simulink model "RadioReceiver_FP_clean"  (R2017a)
settings: Solver=FixedStepDiscrete  StartTime=0.0  StopTime=10.0  RelTol=1e-3
InitFcn:
  | barker = comm.BarkerCode('SamplesPerFrame', 28, 'Length', 11);
  | seq = barker()+1;
  | M = 4;
  | hPSKModTrain   = comm.PSKModulator(M, ...
  |     'PhaseOffset',pi/4, ...
  |     'SymbolMapping','Binary');
  | xPreambleSeq = hPSKModTrain(seq);
  | 
  | 
  | %%%%%%%%%%%%
  | 
  | % AGC Preamble
  | reps = 5;
  | barker = comm.BarkerCode('SamplesPerFrame', 16, 'Length', 13);
  | seq = barker()+1;
  | %preamble = zeros(16*reps,1);
  | preambleFull = repmat(seq,reps,1);
  | rctFilt = comm.RaisedCosineTransmitFilter('FilterSpanInSymbols', 128,...
  | 'RolloffFactor',0.5,...
  | 'OutputSamplesPerSymbol',4);
  | preambleFullFilt = rctFilt(preambleFull);
  | 
  | %%%%%%%%%%%%
  | 
  | RadioSampleRate = 1e6;
  | RadioFrameLength = 1e5;
  | 
  | VibertiTracebackLength = 34+20;
  | numTrainingSamples = 250;
  | crc32Poly = [1 0 0 0 0 0 1 0 0 1 1 0 0 0 0 0 1 0 0 0 1 1 1 0 1 1 0 1 1 0 1 1 1];
  | crcDecodeLag = length(crc32Poly)+2;
  | 
  | %%%%%%%%%%%%
  | 
  | beta = 0.5;
  | span = 8;
  | sps = 4;
  | filterGain = 1;
  | coeff = rcosdesign(beta, span, sps, 'sqrt')*filterGain;
  | 
  | %%%%%%%%%%%%
  | 
  | samplesPerSymbol = 4;
  | maxPacketBits = 8*1500;
  | bItsPerSymbol = 2;
  | CodeRate = 2;
  | tailSymbols = 40;
  | maxPayloadSymbols = maxPacketBits*CodeRate/bItsPerSymbol+tailSymbols;
undefined symbols (not defined in the file or in its folder): F, j
libraries: dsphdlfiltering x20, simulink x7, dspstat3 x2, hdlsllib x2, commdigbbndpm3 x2, commsource2 x1, commcrc2 x1, commseqgen3 x1, commcnvcod2 x1, commutil2 x1, zc706fmc234_lib x1
(part 1 of 3)
settings Model: DataTypeOverride=Off  MinMaxOverflowLogging=MinMaxAndOverflow  FPTRunName=NoOverride  Creator=tcollins  LastModifiedBy=tcollins
settings DataIOCC: SaveOutput=off  SaveTime=off
settings OptimizationCC: BlockReduction=off  ConditionallyExecuteInputs=off  DefaultParameterBehavior=Inlined
settings DebuggingCC: AlgebraicLoopMsg=error  SingleTaskRateTransMsg=error
settings HardwareCC: ProdBitPerPointer=32  ProdBitPerSizeT=32  ProdBitPerPtrDiffT=32  ProdLargestAtomicFloat=None  ProdIntDivRoundTo=Undefined  ProdEndianess=Unspecified  ProdWordSize=32  ProdHWDeviceType=ASIC/FPGA->ASIC/FPGA  ProdEqTarget=off

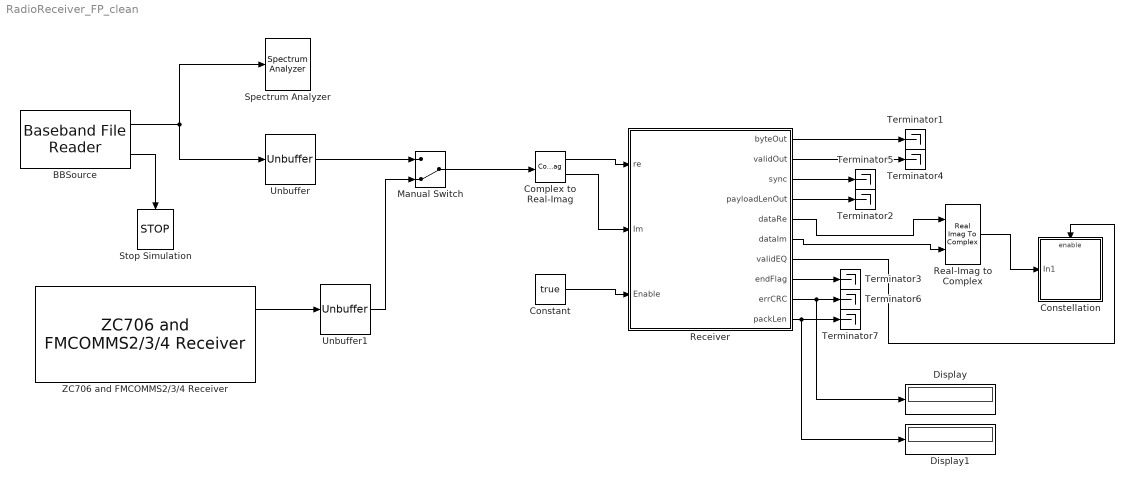
== system RadioReceiver_FP_clean ==
  BBSource : commsource2/Baseband File Reader  Filename=Pluto_1kHz_off.bb  InheritSampleTimeFromFile=on  SampleTime=1  SamplesPerFrame=100000  CyclicRepetition=off  FileEndOutputPort=on  SimulateUsing=Code generation
      settings: SourceProductName=Communications System Toolbox  SourceProductBaseCode=CM
  Complex to Real-Imag : ComplexToRealImag
  Constant : Constant  Value=true  SampleTime=1/RadioSampleRate
  Constellation : Subsystem
  Display : Display
  Display1 : Display
  Manual Switch : ManualSwitch  CurrentSetting=0
  Real-Imag to Complex : RealImagToComplex
  Receiver : Subsystem  TreatAsAtomicUnit=on
  Spectrum Analyzer : SpectrumAnalyzer
  Stop Simulation : Stop
  Terminator{1..7} (7 alike) : Terminator
  Unbuffer : Unbuffer
  Unbuffer1 : Unbuffer
  ZC706 and FMCOMMS2/3/4 Receiver : zc706fmc234_lib/ZC706 and  FMCOMMS2//3//4  Receiver  IPAddress=192.168.3.2  CenterFrequencySource=Dialog  CenterFrequency=2.4e9  GainSource=AGC Slow Attack  Gain=1  ChannelMapping=1  BasebandSampleRate=1e6  EnableBurstMode=on  NumFramesInBurst=10  OutputDataType=int16  SamplesPerFrame=1e6  LostSamplesOutputPort=off  RSSIOutputPort=off  DMATimeoutValue=1  blockMode=Normal  SimulateUsing=Code generation  EnableQuadratureTracking=on  EnableRFDCTracking=on  EnableBasebandDCTracking=on  BypassUserLogic=on  ShowAdvancedProperties=on  ShowInternalProperties=off  subDeviceList=zynqReceiver  sdrExecutionMode=HW  dataUDPPort=-1  ctrlUDPPort=-1  SourceSelect=RF data  SourceConfiguration1=1023  FIRCoefficientSize=[128;128]  FIRCoefficients=[55 -54 42 -126 -123 -317 -399 -581 -646 -711 -634 -507 -263 -10 255 424 492 401 201 -84 -352 -540 -566 -423 -126 234 562 738 701 429 -5 -490 -866 -1007 -834 -372 266 891 1301 1334 936 178 -733 -1524 -1917 -1731 -944 274 1590 2585 2881 2255 741 -1344 -3435 -4850 -4942 -3285 197 5169 10923 16509 20932 23375 23375 20932 16509 10923 5169 197 -3285 -4942 -4850 -3435 -1344 741 2255 2881 2585 1590 274 -944 -1731 -1917 -1524 -733 178 936 1334 1301 891 266 -372 -834 -1007 -866 -490 -5 429 701 738 562 234 -126 -423 -566 -540 -352 -84 201 401 492 424 255 -10 -263 -507 -634 -711 -646 -581 -399 -317 -123 -126 42 -54 55;190 -88 329 -40 239 -99 -24 -349 -377 -611 -573 -604 -395 -229 66 239 394 350 227 -46 -300 -534 -593 -506 -221 137 512 737 765 526 103 -420 -852 -1069 -947 -512 156 841 1341 1450 1100 333 -638 -1531 -2028 -1922 -1152 115 1544 2677 3099 2535 997 -1205 -3479 -5095 -5345 -3750 -199 4965 11002 16895 21580 24172 24172 21580 16895 11002 4965 -199 -3750 -5345 -5095 -3479 -1205 997 2535 3099 2677 1544 115 -1152 -1922 -2028 -1531 -638 333 1100 1450 1341 841 156 -512 -947 -1069 -852 -420 103 526 765 737 512 137 -221 -506 -593 -534 -300 -46 227 350 394 239 66 -229 -395 -604 -573 -611 -377 -349 -24 -99 239 -40 329 -88 190]  FIRGain=[0;-12]  FIRDecimInterpFactor=[4;4]  AnalogFilterCutoff=[3152524;3161715]  FilterPathRates=[983040000 122880000 61440000 30720000 15360000 3840000;983040000 122880000 61440000 30720000 15360000 3840000]  FilterDesignTypeForTx=DefaultFilterFromOther  FilterDesignTypeForRx=DefaultFilter  BISTLoopbackConfig=No Loopback  BISTPRBSMode=PRBS Disable  BISTToneMode=Tone Disable  BISTToneFrequency=F/32  BISTToneLevel=-6  BISTChannelMask=0  DataIsComplex=on
      settings: SourceProductName=Communications System Toolbox Support Package for Xilinx Zynq-Based Radio
  wires:
  BBSource/1 -> Unbuffer/1, Spectrum Analyzer/1
  Constant/1 -> Receiver/3(Enable)
  Complex to Real-Imag/1 -> Receiver/1(re)
  Complex to Real-Imag/2 -> Receiver/2(Im)
  BBSource/2 -> Stop Simulation/1
  Receiver/3(sync) -> Terminator5/1
  Receiver/2(validOut) -> Terminator4/1
  Receiver/1(byteOut) -> Terminator1/1
  Receiver/5(dataRe) -> Real-Imag to Complex/1
  Receiver/6(dataIm) -> Real-Imag to Complex/2
  Real-Imag to Complex/1 -> Constellation/1(In1)
  Receiver/7(validEQ) -> Constellation/Enable
  Receiver/4(payloadLenOut) -> Terminator2/1
  Unbuffer/1 -> Manual Switch/1
  Manual Switch/1 -> Complex to Real-Imag/1
  Unbuffer1/1 -> Manual Switch/2
  ZC706 and FMCOMMS2/3/4 Receiver/1 -> Unbuffer1/1
  Receiver/8(endFlag) -> Terminator3/1
  Receiver/9(errCRC) -> Display/1, Terminator6/1
  Receiver/10(packLen) -> Display1/1, Terminator7/1

== system RadioReceiver_FP_clean/Constellation ==
  In1 : Inport
  Enable : EnablePort
  Constellation Diagram : ConstellationDiagram
  wires:
  In1/1 -> Constellation Diagram/1

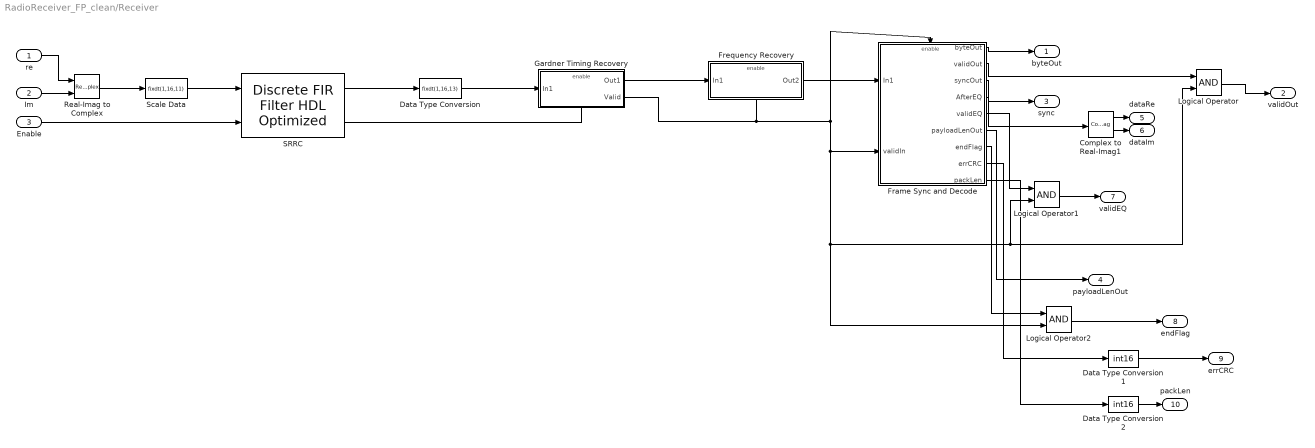
== system RadioReceiver_FP_clean/Receiver ==
  re : Inport
  Im : Inport  Port=2
  Enable : Inport  Port=3
  Complex to Real-Imag1 : ComplexToRealImag
  Data Type Conversion : DataTypeConversion  OutDataTypeStr=fixdt(1,16,13)
  Data Type Conversion1 : DataTypeConversion  OutDataTypeStr=int16
  Data Type Conversion2 : DataTypeConversion  OutDataTypeStr=int16
  Frame Sync and Decode : Subsystem  TreatAsAtomicUnit=on
  Frequency Recovery : Subsystem
  Gardner Timing Recovery : Subsystem
  Logical Operator : Logic  AllPortsSameDT=off  OutDataTypeStr=boolean
  Logical Operator1 : Logic  AllPortsSameDT=off  OutDataTypeStr=boolean
  Logical Operator2 : Logic  AllPortsSameDT=off  OutDataTypeStr=boolean
  Real-Imag to Complex : RealImagToComplex
  SRRC : dsphdlfiltering/Discrete FIR Filter HDL Optimized  Numerator=coeff  Sharing=off  SharingFactor=2  SimulateUsing=Code generation  roundingMode=Floor  overflowMode=on  CoefficientsDataTypeStr=Inherit: Same word length as input  CoefficientsMin=[]  CoefficientsMax=[]  OutputDataTypeStr=fixdt(1,16,11)  OutputMin=[]  OutputMax=[]  ValidInPort=on  ReadyPort=off
      settings: SourceProductName=DSP System Toolbox  SourceProductBaseCode=DS
  Scale Data : DataTypeConversion  OutDataTypeStr=fixdt(1,16,11)  ConvertRealWorld=Stored Integer (SI)  SaturateOnIntegerOverflow=on
  byteOut : Outport
  validOut : Outport  Port=2
  sync : Outport  Port=3
  payloadLenOut : Outport  Port=4
  dataRe : Outport  Port=5
  dataIm : Outport  Port=6
  validEQ : Outport  Port=7
  endFlag : Outport  Port=8
  errCRC : Outport  Port=9
  packLen : Outport  Port=10
  wires:
  Scale Data/1 -> SRRC/1
  SRRC/1 -> Data Type Conversion/1
  Enable/1 -> SRRC/2
  Real-Imag to Complex/1 -> Scale Data/1
  re/1 -> Real-Imag to Complex/1
  Im/1 -> Real-Imag to Complex/2
  SRRC/2 -> Gardner Timing Recovery/Enable
  Data Type Conversion/1 -> Gardner Timing Recovery/1(In1)
  Gardner Timing Recovery/1(Out1) -> Frequency Recovery/1(In1)
  Frequency Recovery/1(Out2) -> Frame Sync and Decode/1(In1)
  Gardner Timing Recovery/2(Valid) -> Logical Operator2/2, Logical Operator1/2, Logical Operator/2, Frame Sync and Decode/2(validIn), Frame Sync and Decode/Enable, Frequency Recovery/Enable
  Frame Sync and Decode/4(AfterEQ) -> Complex to Real-Imag1/1
  Complex to Real-Imag1/1 -> dataRe/1
  Complex to Real-Imag1/2 -> dataIm/1
  Frame Sync and Decode/3(syncOut) -> sync/1
  Frame Sync and Decode/1(byteOut) -> byteOut/1
  Frame Sync and Decode/2(validOut) -> Logical Operator/1
  Logical Operator/1 -> validOut/1
  Logical Operator1/1 -> validEQ/1
  Frame Sync and Decode/5(validEQ) -> Logical Operator1/1
  Frame Sync and Decode/6(payloadLenOut) -> payloadLenOut/1
  Frame Sync and Decode/8(errCRC) -> Data Type Conversion1/1
  Frame Sync and Decode/9(packLen) -> Data Type Conversion2/1
  Frame Sync and Decode/7(endFlag) -> Logical Operator2/1
  Data Type Conversion1/1 -> errCRC/1
  Logical Operator2/1 -> endFlag/1
  Data Type Conversion2/1 -> packLen/1

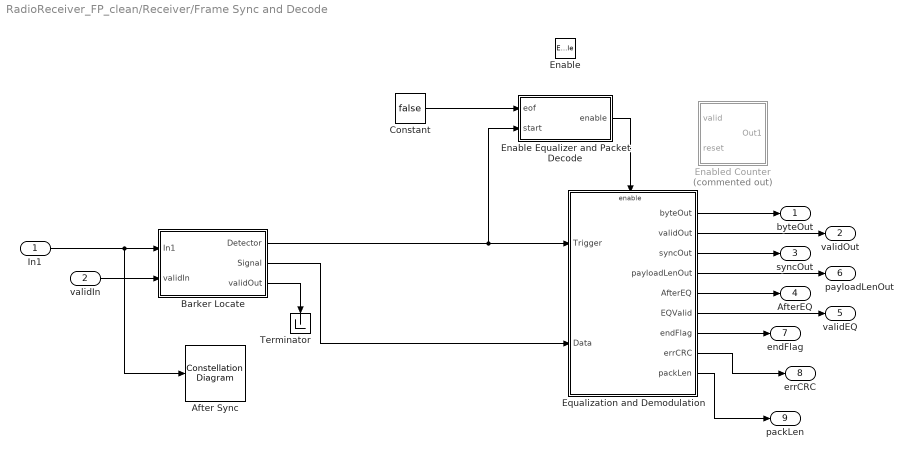
== system RadioReceiver_FP_clean/Receiver/Frame Sync and Decode ==
  In1 : Inport
  validIn : Inport  Port=2
  Enable : EnablePort
  After Sync : ConstellationDiagram
  Barker Locate : Subsystem  mask{Threshold=0.75}
  Constant : Constant  Value=false  SampleTime=1e-6
  Enable Equalizer and Packet Decode : MATLAB Function  TreatAsAtomicUnit=on
  Enabled Counter : Subsystem  Commented=on
  Equalization and Demodulation : Subsystem
  Terminator : Terminator
  byteOut : Outport  InitialOutput=0
  validOut : Outport  Port=2  InitialOutput=0
  syncOut : Outport  Port=3  InitialOutput=0
  AfterEQ : Outport  Port=4  InitialOutput=0
  validEQ : Outport  Port=5  InitialOutput=0
  payloadLenOut : Outport  Port=6  InitialOutput=0
  endFlag : Outport  Port=7  InitialOutput=0
  errCRC : Outport  Port=8  InitialOutput=0
  packLen : Outport  Port=9  InitialOutput=0
  wires:
  In1/1 -> After Sync/1, Barker Locate/1(In1)
  Equalization and Demodulation/6(EQValid) -> validEQ/1
  Equalization and Demodulation/5(AfterEQ) -> AfterEQ/1
  validIn/1 -> Barker Locate/2(validIn)
  Enable Equalizer and Packet Decode/1(enable) -> Equalization and Demodulation/Enable
  Constant/1 -> Enable Equalizer and Packet Decode/1(eof)
  Barker Locate/3(validOut) -> Terminator/1
  Barker Locate/1(Detector) -> Enable Equalizer and Packet Decode/2(start), Equalization and Demodulation/1(Trigger)
  Barker Locate/2(Signal) -> Equalization and Demodulation/2(Data)
  Equalization and Demodulation/1(byteOut) -> byteOut/1
  Equalization and Demodulation/2(validOut) -> validOut/1
  Equalization and Demodulation/3(syncOut) -> syncOut/1
  Equalization and Demodulation/4(payloadLenOut) -> payloadLenOut/1
  Equalization and Demodulation/7(endFlag) -> endFlag/1
  Equalization and Demodulation/8(errCRC) -> errCRC/1
  Equalization and Demodulation/9(packLen) -> packLen/1

== system RadioReceiver_FP_clean/Receiver/Frequency Recovery ==
  note: Max Phase Lock Delay= 1.3/(NormLoopBandwidth*SampleRate)
  note: Frequency Lock Delay = SampleRate*4*NormalizedPullInRange^2)/ (SampleRate*NormLoopBandwidth)^3;
  note: Pull in range (Hz) = 2*pi*sqrt(2)*DampingFactor*NormLoopBandwidth*SampleRate
  In1 : Inport
  Enable : EnablePort
  Data Type Conversion : DataTypeConversion  OutDataTypeStr=fixdt(1,16,10)
  Delay : Delay  DelayLength=1
  Loop Filter : Subsystem  mask{BnTs=0.1, zeta=2*1/sqrt(2), N=1}
      mask prompts: BnTs "Normalized Loop Bandwidth"; zeta "Damping Factor"; N "Number of Samples/Symbol"
      mask init:
      | % See C.57 to C.61 in Michael Rice's "Digital Communications 
      | % - A Discrete-Time Approach" for details
      | 
      | %theta = BnTs/(zeta+0.25/zeta);  %0.0385
      | %d = 1 + 2*zeta*theta + theta*theta; %1.1938
      | %K1 = zeta*theta/d; %0.0805
      | %K2 = theta*theta/(d*2); %6.1958e-04
      | 
      | %%
      | DampingFactor = zeta;
      | samplesPerSymbol = N;
      | NormalizedLoopBandwidth = BnTs;
      | %
      | PhaseRecoveryLoopBandwidth = NormalizedLoopBandwidth*samplesPerSymbol;
      |  
      | PhaseRecoveryGain = samplesPerSymbol;
      |  
      | PhaseErrorDetectorGain = 1;
      | 
      | 
      | theta = PhaseRecoveryLoopBandwidth/...
      |     ((DampingFactor + 0.25/DampingFactor)*samplesPerSymbol);
      |  
      | d = 1 + 2*DampingFactor*theta + theta*theta;
      |  
      | % K1
      | K1 = (4*DampingFactor*theta/d)/...
      |     (PhaseErrorDetectorGain*PhaseRecoveryGain);
      | % K2
      | K2 = (4/samplesPerSymbol*theta*theta/d)/...
      |     (PhaseErrorDetectorGain*PhaseRecoveryGain);
      mask Display: disp('Loop Filter')
  PED For QPSK : Subsystem
  Phase Shift FP : Subsystem
  State Control : StateControl  StateControl=Synchronous
  Out2 : Outport
  wires:
  Delay/1 -> PED For QPSK/1(In1), Out2/1
  Data Type Conversion/1 -> Loop Filter/1(e)
  Loop Filter/1(v) -> Phase Shift FP/2(Phi)
  In1/1 -> Phase Shift FP/1(In1)
  Phase Shift FP/1(Out1) -> Delay/1
  PED For QPSK/1(Out1) -> Data Type Conversion/1

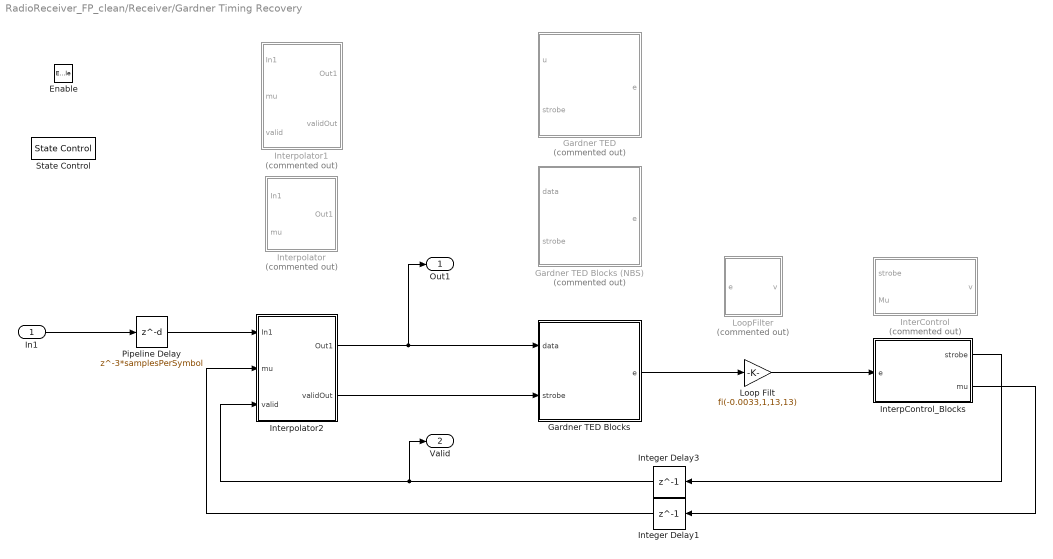
== system RadioReceiver_FP_clean/Receiver/Gardner Timing Recovery ==
  In1 : Inport  OutDataTypeStr=fixdt(1,16,13)
  Enable : EnablePort
  Gardner TED : Subsystem  Commented=on  TreatAsAtomicUnit=on  Variant=on  VariantControl=Variant1  OverrideUsingVariant=false()
  Gardner TED Blocks : Subsystem
  Gardner TED Blocks (NBS) : Subsystem  Commented=on
  Integer Delay1 : Delay  DelayLength=1  InputProcessing=Inherited
  Integer Delay3 : Delay  DelayLength=1  InputProcessing=Inherited
  InterControl : Subsystem  Commented=on  TreatAsAtomicUnit=on  Variant=on  VariantControl=Variant1  OverrideUsingVariant=false()
  InterpControl_Blocks : Subsystem
  Interpolator : Subsystem  Commented=on
  Interpolator1 : Subsystem  Commented=on
  Interpolator2 : Subsystem
  Loop Filt : Gain  Gain=fi(-0.0033,1,13,13)  OutDataTypeStr=fixdt(1,12,16)
  LoopFilter : Subsystem  Commented=on  mask{zeta=sqrt(2), BnTs=0.01, Kp=2.7}
      mask prompts: zeta "DampingFactor"; BnTs "NormalizedLoopBandwidth"; Kp "DetectionGain"
      mask init:
      | K0 = -1;
      | SPS = 4;
      | theta = BnTs/SPS/(zeta + 0.25/zeta);
      | d  = (1 + 2*zeta*theta + theta^2) * K0 * Kp;
      | ProportionalGain = (4*zeta*theta) /d;
      | IntegratorGain   = (4*theta*theta)/d;
  Pipeline Delay : Delay  DelayLength=3*samplesPerSymbol
  State Control : StateControl  StateControl=Synchronous
  Out1 : Outport
      settings: SignalType=complex
  Valid : Outport  Port=2  OutDataTypeStr=boolean
  wires:
  In1/1 -> Pipeline Delay/1
  Integer Delay3/1 -> Interpolator2/3(valid), Valid/1
  Integer Delay1/1 -> Interpolator2/2(mu)
  Pipeline Delay/1 -> Interpolator2/1(In1)
  InterpControl_Blocks/2(mu) -> Integer Delay1/1
  InterpControl_Blocks/1(strobe) -> Integer Delay3/1
  Gardner TED Blocks/1(e) -> Loop Filt/1
  Loop Filt/1 -> InterpControl_Blocks/1(e)
  Interpolator2/2(validOut) -> Gardner TED Blocks/2(strobe)
  Interpolator2/1(Out1) -> Gardner TED Blocks/1(data), Out1/1

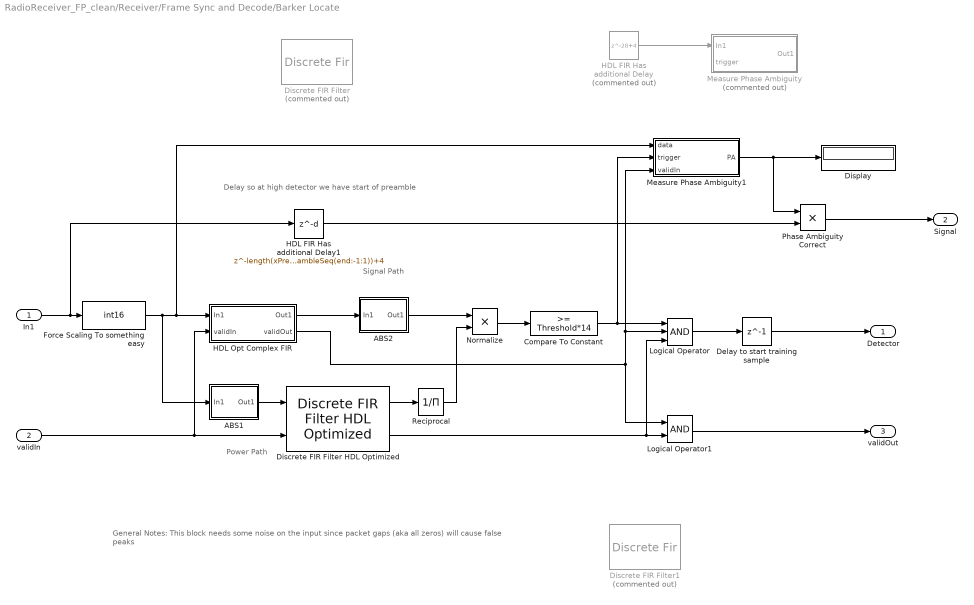
== system RadioReceiver_FP_clean/Receiver/Frame Sync and Decode/Barker Locate ==
  note: General Notes:
      | This block needs some noise on the input since packet gaps (aka all zeros) will cause false peaks
  note: Delay so at high detector we have start of preamble
  note: Power Path
  note: Signal Path
  In1 : Inport
  validIn : Inport  Port=2
  ABS1 : Subsystem
  ABS2 : Subsystem
  Compare To Constant : simulink/Logic and Bit Operations/Compare To Constant  relop=>=  const=Threshold*14  OutDataTypeStr=boolean
  "Delay to start training sample " : Delay  DelayLength=1
  Discrete FIR Filter : DiscreteFir  Commented=on  Coefficients=xPreambleSeq(end:-1:1).'  AccumDataTypeStr=Inherit: Same as product output  OutDataTypeStr=int16
  Discrete FIR Filter HDL Optimized : dsphdlfiltering/Discrete FIR Filter HDL Optimized  Numerator=ones(1,length(xPreambleSeq)*1)/1  Sharing=off  SharingFactor=2  SimulateUsing=Code generation  roundingMode=Floor  overflowMode=off  CoefficientsDataTypeStr=Inherit: Same word length as input  CoefficientsMin=[]  CoefficientsMax=[]  OutputDataTypeStr=fixdt(1,17,0)  OutputMin=[]  OutputMax=[]  ValidInPort=on  ReadyPort=off
      settings: SourceProductName=DSP System Toolbox  SourceProductBaseCode=DS
  Discrete FIR Filter1 : DiscreteFir  Commented=on  Coefficients=ones(1,length(xPreambleSeq)*1)/1  AccumDataTypeStr=Inherit: Same as product output  OutDataTypeStr=int16  SaturateOnIntegerOverflow=on
  Display : Display
  Force Scaling To something easy : DataTypeConversion  OutDataTypeStr=int16  SaturateOnIntegerOverflow=on
  HDL FIR Has additional Delay : Delay  Commented=on  DelayLength=28+4
  HDL FIR Has additional Delay1 : Delay  DelayLength=length(xPreambleSeq(end:-1:1))+4
  HDL Opt Complex FIR : Subsystem  mask{Taps=xPreambleSeq(end:-1:1).'}
  Logical Operator : Logic  Inputs=3  AllPortsSameDT=off  OutDataTypeStr=boolean
  Logical Operator1 : Logic  AllPortsSameDT=off  OutDataTypeStr=boolean
  Measure Phase Ambiguity : Subsystem  Commented=on
  Measure Phase Ambiguity1 : Subsystem
  Normalize : Product  Inputs=**  OutDataTypeStr=int16  RndMeth=Simplest  SaturateOnIntegerOverflow=on
  Phase Ambiguity Correct : Product  OutDataTypeStr=fixdt(1,16,14)
  Reciprocal : Product  Inputs=/  SaturateOnIntegerOverflow=on  RndMeth=Zero
  Detector : Outport
  Signal : Outport  Port=2
  validOut : Outport  Port=3
  wires:
  HDL Opt Complex FIR/1(Out1) -> ABS2/1(In1)
  ABS2/1(Out1) -> Normalize/1
  "Delay to start training sample "/1 -> Detector/1
  Normalize/1 -> Compare To Constant/1
  In1/1 -> HDL FIR Has additional Delay1/1, Force Scaling To something easy/1
  ABS1/1(Out1) -> Discrete FIR Filter HDL Optimized/1
  Logical Operator/1 -> "Delay to start training sample "/1
  Logical Operator1/1 -> validOut/1
  Measure Phase Ambiguity1/1(PA) -> Display/1, Phase Ambiguity Correct/1
  validIn/1 -> HDL Opt Complex FIR/2(validIn), Discrete FIR Filter HDL Optimized/2
  Discrete FIR Filter HDL Optimized/2 -> Logical Operator1/2, Logical Operator/3
  HDL Opt Complex FIR/2(validOut) -> Logical Operator1/1, Measure Phase Ambiguity1/3(validIn), Logical Operator/2
  Phase Ambiguity Correct/1 -> Signal/1
  HDL FIR Has additional Delay1/1 -> Phase Ambiguity Correct/2
  Force Scaling To something easy/1 -> ABS1/1(In1), HDL Opt Complex FIR/1(In1), Measure Phase Ambiguity1/1(data)
  Compare To Constant/1 -> Measure Phase Ambiguity1/2(trigger), Logical Operator/1
  HDL FIR Has additional Delay/1 -> Measure Phase Ambiguity/1(In1)
  Discrete FIR Filter HDL Optimized/1 -> Reciprocal/1
  Reciprocal/1 -> Normalize/2

== system RadioReceiver_FP_clean/Receiver/Frame Sync and Decode/Enabled Counter ==
  valid : Inport
  reset : Inport  Port=2
  Compare To Constant : simulink/Logic and Bit Operations/Compare To Constant  relop=<  const=maxPayloadSymbols  OutDataTypeStr=boolean
  HDL Counter : hdlsllib/HDL Operations/HDL Counter  CountType=Count limited  CountInit=maxPayloadSymbols  CountStep=1  CountMax=maxPayloadSymbols  CountFromType=Specify  CountFrom=0  CountResetPort=on  CountLoadPort=off  CountEnbPort=on  CountDirPort=off  CountDataType=Unsigned  CountWordLen=32  CountFracLen=0  CountSampTime=1
      settings: SourceProductName=HDL Coder  SourceProductBaseCode=HD
  Logical Operator : Logic  AllPortsSameDT=off  OutDataTypeStr=boolean
  Out1 : Outport
  wires:
  valid/1 -> Logical Operator/2, HDL Counter/2
  reset/1 -> HDL Counter/1
  HDL Counter/1 -> Compare To Constant/1
  Logical Operator/1 -> Out1/1
  Compare To Constant/1 -> Logical Operator/1

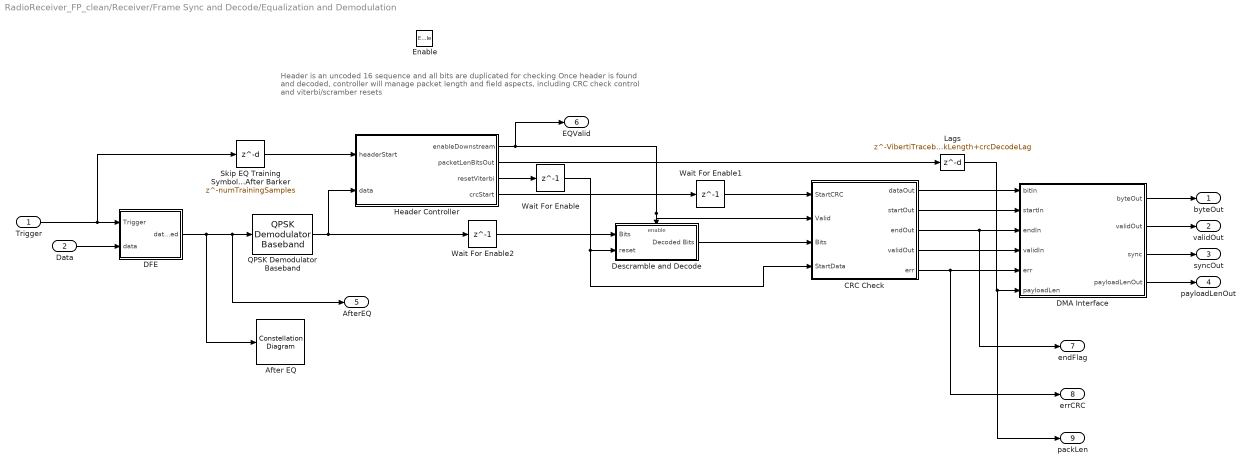
== system RadioReceiver_FP_clean/Receiver/Frame Sync and Decode/Equalization and Demodulation ==
  note: Header is an uncoded 16 sequence and all bits are duplicated for checking
      |
      | Once header is found and decoded, controller will manage packet length and field aspects,
      | including CRC check control and viterbi/scramber resets
  Trigger : Inport
  Data : Inport  Port=2
  Enable : EnablePort
  After EQ : ConstellationDiagram
  CRC Check : Subsystem
  DFE : Subsystem
  DMA Interface : Subsystem
  Descramble and Decode : Subsystem  TreatAsAtomicUnit=on
  Header Controller : MATLAB Function  TreatAsAtomicUnit=on
  Lags : Delay  DelayLength=VibertiTracebackLength+crcDecodeLag
  QPSK Demodulator Baseband : commdigbbndpm3/QPSK Demodulator Baseband  OutType=Bit  DecType=Hard decision  VarSource=Dialog  Variance=1  Dec=Binary  Ph=pi/4  outDtype1=boolean  outDtype2=Inherit via internal rule  derotateFactorWordLen=16  derotateFactorDataTypeStr=Inherit: Same word length as input  derotateFactorLastDataTypeStr=Inherit: Same word length as input
  Skip EQ Training Symbols After Barker : Delay  DelayLength=numTrainingSamples
  Wait For Enable : Delay  DelayLength=1
  Wait For Enable1 : Delay  DelayLength=1
  Wait For Enable2 : Delay  DelayLength=1
  byteOut : Outport  InitialOutput=0
  validOut : Outport  Port=2  InitialOutput=0
  syncOut : Outport  Port=3  InitialOutput=0
  payloadLenOut : Outport  Port=4  InitialOutput=0
  AfterEQ : Outport  Port=5  InitialOutput=0
  EQValid : Outport  Port=6  InitialOutput=0
  endFlag : Outport  Port=7  InitialOutput=0
  errCRC : Outport  Port=8  InitialOutput=0
  packLen : Outport  Port=9  InitialOutput=0
  wires:
  Skip EQ Training Symbols After Barker/1 -> Header Controller/1(headerStart)
  Data/1 -> DFE/2(data)
  DFE/1(dataEQed) -> AfterEQ/1, QPSK Demodulator Baseband/1, After EQ/1
  QPSK Demodulator Baseband/1 -> Header Controller/2(data), Wait For Enable2/1
  Descramble and Decode/1(Decoded Bits) -> CRC Check/3(Bits)
  Header Controller/1(enableDownstream) -> EQValid/1, CRC Check/2(Valid), Descramble and Decode/Enable
  Header Controller/4(crcStart) -> Wait For Enable1/1
  Header Controller/3(resetViterbi) -> Wait For Enable/1
  Trigger/1 -> Skip EQ Training Symbols After Barker/1, DFE/1(Trigger)
  Wait For Enable/1 -> CRC Check/4(StartData), Descramble and Decode/2(reset)
  Wait For Enable2/1 -> Descramble and Decode/1(Bits)
  Wait For Enable1/1 -> CRC Check/1(StartCRC)
  Header Controller/2(packetLenBitsOut) -> Lags/1
  CRC Check/1(dataOut) -> DMA Interface/1(bitIn)
  CRC Check/2(startOut) -> DMA Interface/2(startIn)
  CRC Check/3(endOut) -> endFlag/1, DMA Interface/3(endIn)
  CRC Check/4(validOut) -> DMA Interface/4(validIn)
  CRC Check/5(err) -> errCRC/1, DMA Interface/5(err)
  Lags/1 -> packLen/1, DMA Interface/6(payloadLen)
  DMA Interface/1(byteOut) -> byteOut/1
  DMA Interface/2(validOut) -> validOut/1
  DMA Interface/3(sync) -> syncOut/1
  DMA Interface/4(payloadLenOut) -> payloadLenOut/1

== system RadioReceiver_FP_clean/Receiver/Frequency Recovery/Loop Filter ==
  note: Proportional-plus-Integrator Loop Filter,
      | Infinite DC Response to guarantee convergence
  e : Inport
  Add1 : Sum  RndMeth=Nearest  OutDataTypeStr=Inherit: Same as first input
  Add2 : Sum  OutDataTypeStr=Inherit: Same as first input
  Delay : Delay  DelayLength=1
  Delay3 : Delay  DelayLength=1
  Delay4 : Delay  DelayLength=1
  Flip Sign : MATLAB Function  Commented=on  TreatAsAtomicUnit=on
  Gain : Gain  Gain=-1.0  OutDataTypeStr=fixdt(1,25,20)
  K1 : Gain  Gain=K2  OutDataTypeStr=Inherit: Same as input
  K2 : Gain  Gain=K1  OutDataTypeStr=Inherit: Same as input
  Sum2 : Sum  OutDataTypeStr=Inherit: Same as first input
  v : Outport
  wires:
  K1/1 -> Sum2/1
  Add1/1 -> Sum2/2
  e/1 -> K2/1, K1/1
  K2/1 -> Delay/1, Add1/2
  Delay/1 -> Add1/1
  Sum2/1 -> Delay3/1
  Delay3/1 -> Add2/1
  Delay4/1 -> Add2/2
  Add2/1 -> Delay4/1, Flip Sign/1(u), Gain/1
  Gain/1 -> v/1

== system RadioReceiver_FP_clean/Receiver/Frequency Recovery/PED For QPSK ==
  In1 : Inport
  Complex to Real-Imag : ComplexToRealImag
  Product : Product
  Product1 : Product
  Sign : Signum
  Sign1 : Signum
  Subtract : Sum  Inputs=+-
  Out1 : Outport
  wires:
  In1/1 -> Complex to Real-Imag/1
  Complex to Real-Imag/1 -> Product1/1, Sign/1
  Complex to Real-Imag/2 -> Product/2, Sign1/1
  Sign/1 -> Product/1
  Sign1/1 -> Product1/2
  Product/1 -> Subtract/1
  Product1/1 -> Subtract/2
  Subtract/1 -> Out1/1

== system RadioReceiver_FP_clean/Receiver/Frequency Recovery/Phase Shift FP ==
  In1 : Inport
  Phi : Inport  Port=2
  Complex Phase Shift : commutil2/Complex Phase Shift  Commented=on
      settings: SourceProductName=Communications System Toolbox  SourceProductBaseCode=CM
  Cosine HDL Optimized : hdlsllib/Lookup Tables/Cosine HDL Optimized  OutputFormula=exp(j*2*pi*u)  NumDataPoints=256  TableDataTypeStr=fixdt(0,32,22)  SimulateLUTROMDelay=off
      settings: SourceProductName=HDL Coder  SourceProductBaseCode=HD
  Data Type Conversion1 : DataTypeConversion  Commented=on  OutDataTypeStr=double
  Data Type Conversion2 : DataTypeConversion  Commented=on  OutDataTypeStr=double
  Data Type Conversion3 : DataTypeConversion  Commented=on  OutDataTypeStr=fixdt(1,16,13)
  Gain : Gain  Gain=1/(2*pi)  ParamDataTypeStr=fixdt(1,25,20)  OutDataTypeStr=fixdt(1,25,20)  SaturateOnIntegerOverflow=on
  Product : Product  OutDataTypeStr=fixdt(1,16,13)  SaturateOnIntegerOverflow=on
  Out1 : Outport
  wires:
  Product/1 -> Out1/1
  Cosine HDL Optimized/1 -> Product/2
  In1/1 -> Data Type Conversion2/1, Product/1
  Phi/1 -> Data Type Conversion1/1, Gain/1
  Gain/1 -> Cosine HDL Optimized/1
  Complex Phase Shift/1 -> Data Type Conversion3/1
  Data Type Conversion2/1 -> Complex Phase Shift/1
  Data Type Conversion1/1 -> Complex Phase Shift/2

== system RadioReceiver_FP_clean/Receiver/Gardner Timing Recovery/Gardner TED ==
  note: This variant subsystem was automatically generated by the Fixed-Point Tool to convert a MATLAB function block to fixed-point.
      |
      | The variant subsystem contains two blocks:
      | 1. Gardner TED is the original code from the MATLAB function block. Modify this block to update your code or resolve errors.
      |
      | 2. Gardner TED_FixPt is the generated fixed-point code for the MATLAB function block. Any modifications to this block will be overwritten on the next conversion.
      |
      | The Fixed-Point Tool will select an appropriate variant based on the Model Settings. Learn more. .
  "u " : Inport
  "strobe " : Inport  Port=2
  Gardner TED : MATLAB Function  TreatAsAtomicUnit=on  VariantControl=false()
  Gardner TED_FixPt : MATLAB Function  TreatAsAtomicUnit=on  VariantControl=(default)
  " e" : Outport

== system RadioReceiver_FP_clean/Receiver/Gardner Timing Recovery/Gardner TED Blocks ==
  note: This is for QPSK and 4 SamplesPerSymbol ONLY
  data : Inport
  strobe : Inport  Port=2
  Add : Sum  OutDataTypeStr=fixdt(1,16,11)
  Check Only Strobe Condition : simulink/Logic and Bit Operations/Compare To Constant  relop===  const=uint8(1)  OutDataTypeStr=boolean
  Complex to Real-Imag : ComplexToRealImag
  Constant : Constant  Value=0  OutDataTypeStr=fixdt(1,16,11)  SampleTime=1e-6
  Imag Error : Subsystem
  Logical Operator : Logic  AllPortsSameDT=off  OutDataTypeStr=boolean
  Map [0,1,2,3] to [0,1,2,2] : LookupNDDirect  NumberOfTableDimensions=1  Table=[0 1 2 2]  DiagnosticForOutOfRangeInput=Error  TableDataTypeStr=uint8
  Real Error : Subsystem
  Strobe Buffer1 : simulink/Discrete/Tapped Delay  vinit=0.0  samptime=-1  NumDelays=samplesPerSymbol-1  DelayOrder=Oldest  includeCurrent=on
  Sum of Elements1 : Sum  Inputs=+  OutDataTypeStr=int8
  Switch : Switch  Criteria=u2 ~= 0
  e : Outport
  wires:
  Switch/1 -> e/1
  strobe/1 -> Strobe Buffer1/1, Logical Operator/2
  Complex to Real-Imag/2 -> Imag Error/1(data)
  Sum of Elements1/1 -> Check Only Strobe Condition/1, Map [0,1,2,3] to [0,1,2,2]/1
  Check Only Strobe Condition/1 -> Logical Operator/1
  Constant/1 -> Switch/3
  Complex to Real-Imag/1 -> Real Error/1(data)
  data/1 -> Complex to Real-Imag/1
  Map [0,1,2,3] to [0,1,2,2]/1 -> Imag Error/2(strobe sum), Real Error/2(strobe sum)
  Strobe Buffer1/1 -> Sum of Elements1/1
  Real Error/1(Out1) -> Add/1
  Imag Error/1(Out1) -> Add/2
  Add/1 -> Switch/1
  Logical Operator/1 -> Switch/2

== system RadioReceiver_FP_clean/Receiver/Gardner Timing Recovery/Gardner TED Blocks (NBS) ==
  note: This is for QPSK and 4 SamplesPerSymbol ONLY
  data : Inport
  strobe : Inport  Port=2
  Add : Sum  OutDataTypeStr=fixdt(1,16,11)
  Complex to Real-Imag : ComplexToRealImag
  Constant : Constant  Value=0  OutDataTypeStr=fixdt(1,16,11)  SampleTime=1e-6
  Constant1 : Constant  Value=uint8(1)  SampleTime=1e-06
  Imag Error : Subsystem
  Logical Operator : Logic  AllPortsSameDT=off  OutDataTypeStr=boolean
  Logical Operator1 : Logic  Operator=OR  Inputs=1  IconShape=distinctive  AllPortsSameDT=off  OutDataTypeStr=boolean
  Real Error : Subsystem
  Strobe Buffer1 : simulink/Discrete/Tapped Delay  vinit=0.0  samptime=-1  NumDelays=samplesPerSymbol-1  DelayOrder=Oldest  includeCurrent=off
  Switch : Switch
  e : Outport
  wires:
  Switch/1 -> e/1
  strobe/1 -> Strobe Buffer1/1, Logical Operator/2
  Complex to Real-Imag/2 -> Imag Error/1(data)
  Imag Error/1(Out1) -> Add/2
  Add/1 -> Switch/1
  Logical Operator1/1 -> Logical Operator/1
  Logical Operator/1 -> Switch/2
  Constant/1 -> Switch/3
  Complex to Real-Imag/1 -> Real Error/1(data)
  Real Error/1(Out1) -> Add/1
  data/1 -> Complex to Real-Imag/1
  Constant1/1 -> Imag Error/2(strobe sum), Real Error/2(strobe sum)
  Strobe Buffer1/1 -> Logical Operator1/1

== system RadioReceiver_FP_clean/Receiver/Gardner Timing Recovery/InterControl ==
  note: This variant subsystem was automatically generated by the Fixed-Point Tool to convert a MATLAB function block to fixed-point.
      |
      | The variant subsystem contains two blocks:
      | 1. InterControl is the original code from the MATLAB function block. Modify this block to update your code or resolve errors.
      |
      | 2. InterControl_FixPt is the generated fixed-point code for the MATLAB function block. Any modifications to this block will be overwritten on the next conversion.
      |
      | The Fixed-Point Tool will select an appropriate variant based on the Model Settings. Learn more. .
  "v " : Inport
  InterControl : MATLAB Function  TreatAsAtomicUnit=on  VariantControl=false()
  InterControl_FixPt : MATLAB Function  TreatAsAtomicUnit=on  VariantControl=(default)
  " strobe" : Outport
  " Mu" : Outport  Port=2

== system RadioReceiver_FP_clean/Receiver/Gardner Timing Recovery/InterpControl_Blocks ==
  e : Inport
  1/W : Constant  Value=fi(1/samplesPerSymbol,0,16,14)  SampleTime=1e-6
  Add : Sum  OutDataTypeStr=fixdt(0,15,15)
  Calculate New mu : Subsystem
  NCOCounter State : Delay  DelayLength=1  InitialCondition=fi(0,0,16,16)
  Subtract1 : Sum  Inputs=-+  OutDataTypeStr=fixdt(0,15,15)
  Update mu on strobe : Switch  Criteria=u2 > Threshold
  saved mu : Delay  DelayLength=1
  strobe == W>NCOCounter : RelationalOperator  Operator=>  OutDataTypeStr=boolean  RndMeth=Nearest
  strobe : Outport
  mu : Outport  Port=2
  wires:
  strobe == W>NCOCounter/1 -> Update mu on strobe/2, strobe/1
  Update mu on strobe/1 -> mu/1, saved mu/1
  saved mu/1 -> Update mu on strobe/3
  Calculate New mu/1(mu) -> Update mu on strobe/1
  e/1 -> Add/1
  1/W/1 -> Add/2
  NCOCounter State/1 -> Calculate New mu/2(NCOCounter), strobe == W>NCOCounter/2, Subtract1/2
  Subtract1/1 -> NCOCounter State/1
  Add/1 -> Calculate New mu/1(W), strobe == W>NCOCounter/1, Subtract1/1

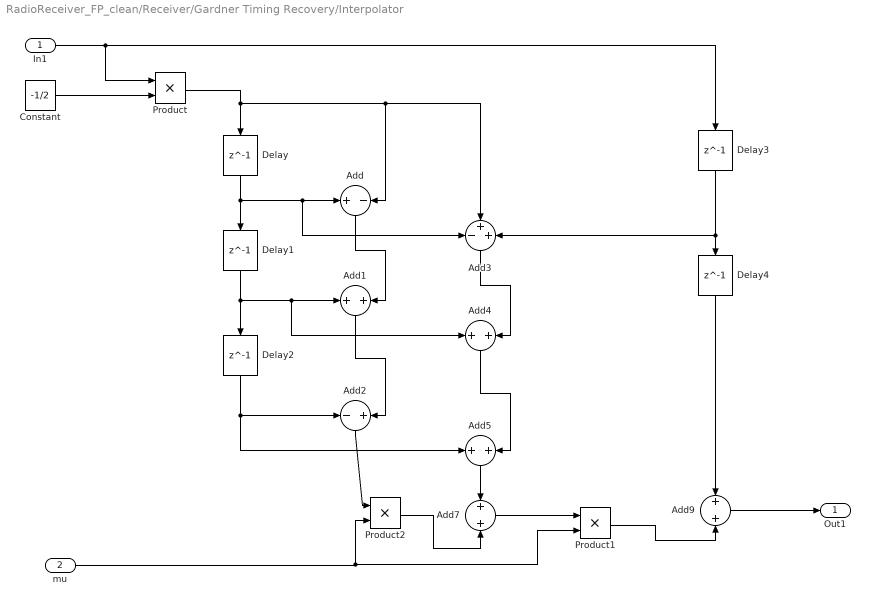
== system RadioReceiver_FP_clean/Receiver/Gardner Timing Recovery/Interpolator ==
  In1 : Inport  OutDataTypeStr=fixdt(1,16,13)
  mu : Inport  Port=2  OutDataTypeStr=fixdt(0,16,16)
  Add : Sum  Inputs=+-  OutDataTypeStr=fixdt(1,16,15)
  Add{1,4..5,7} (4 alike) : Sum  OutDataTypeStr=fixdt(1,16,14)
  Add2 : Sum  Inputs=-+  OutDataTypeStr=fixdt(1,16,15)
  Add3 : Sum  Inputs=-++  OutDataTypeStr=fixdt(1,16,13)
  Add9 : Sum  OutDataTypeStr=fixdt(1,16,13)
  Constant : Constant  Value=-1/2  OutDataTypeStr=fixdt(1,16,16)  SampleTime=1e-06
  Delay{,1..4} (5 alike) : Delay  DelayLength=1
  Product : Product  OutDataTypeStr=fixdt(1,16,14)
  Product1 : Product  OutDataTypeStr=fixdt(1,16,14)
  Product2 : Product  OutDataTypeStr=fixdt(1,16,15)
  Out1 : Outport
  wires:
  In1/1 -> Delay3/1, Product/1
  Constant/1 -> Product/2
  Product/1 -> Add3/2, Add/2, Delay/1
  Delay/1 -> Add3/1, Add/1, Delay1/1
  Delay1/1 -> Add4/1, Add1/1, Delay2/1
  Add/1 -> Add1/2
  Delay2/1 -> Add5/1, Add2/1
  Add1/1 -> Add2/2
  Add3/1 -> Add4/2
  Add4/1 -> Add5/2
  Add2/1 -> Product2/1
  mu/1 -> Product2/2, Product1/2
  Add5/1 -> Add7/1
  Product2/1 -> Add7/2
  Add9/1 -> Out1/1
  Delay3/1 -> Add3/3, Delay4/1
  Delay4/1 -> Add9/1
  Add7/1 -> Product1/1
  Product1/1 -> Add9/2

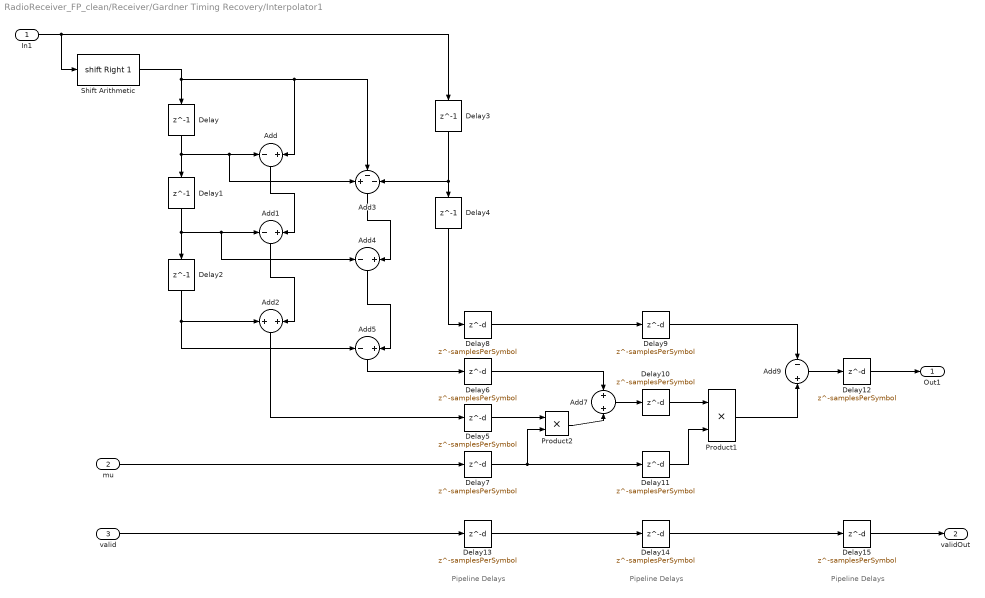
== system RadioReceiver_FP_clean/Receiver/Gardner Timing Recovery/Interpolator1 ==
  note: Pipeline Delays
  note: Pipeline Delays
  note: Pipeline Delays
  In1 : Inport  OutDataTypeStr=fixdt(1,16,13)
  mu : Inport  Port=2  OutDataTypeStr=fixdt(0,14,15)
  valid : Inport  Port=3  OutDataTypeStr=boolean
  Add : Sum  Inputs=-+  OutDataTypeStr=fixdt(1,16,15)
  Add1 : Sum  Inputs=-+  OutDataTypeStr=fixdt(1,16,14)
  Add2 : Sum  OutDataTypeStr=fixdt(1,16,15)
  Add3 : Sum  Inputs=+--  OutDataTypeStr=fixdt(1,16,13)
  Add4 : Sum  Inputs=-+  OutDataTypeStr=fixdt(1,16,14)
  Add5 : Sum  Inputs=-+  OutDataTypeStr=fixdt(1,16,14)
  Add7 : Sum  OutDataTypeStr=fixdt(1,16,14)
  Add9 : Sum  Inputs=-+  OutDataTypeStr=fixdt(1,16,13)
  Delay{,1..4} (5 alike) : Delay  DelayLength=1
  Delay{5..15} (11 alike) : Delay  DelayLength=samplesPerSymbol
  Product1 : Product  OutDataTypeStr=fixdt(1,16,14)
  Product2 : Product  OutDataTypeStr=fixdt(1,16,15)
  Shift Arithmetic : ArithShift  BitShiftNumber=1  BitShiftDirection=Right
  Out1 : Outport
  validOut : Outport  Port=2
  wires:
  In1/1 -> Delay3/1, Shift Arithmetic/1
  Shift Arithmetic/1 -> Add3/2, Add/2, Delay/1
  Delay/1 -> Add3/1, Add/1, Delay1/1
  Delay1/1 -> Add4/1, Add1/1, Delay2/1
  Add/1 -> Add1/2
  Delay2/1 -> Add5/1, Add2/1
  Add1/1 -> Add2/2
  Add3/1 -> Add4/2
  Add4/1 -> Add5/2
  Add2/1 -> Delay5/1
  mu/1 -> Delay7/1
  Add5/1 -> Delay6/1
  Product2/1 -> Add7/2
  Add9/1 -> Delay12/1
  Delay3/1 -> Add3/3, Delay4/1
  Delay4/1 -> Delay8/1
  Product1/1 -> Add9/2
  Delay5/1 -> Product2/1
  Delay6/1 -> Add7/1
  Delay7/1 -> Product2/2, Delay11/1
  Delay8/1 -> Delay9/1
  Delay9/1 -> Add9/1
  Add7/1 -> Delay10/1
  Delay10/1 -> Product1/1
  Delay11/1 -> Product1/2
  valid/1 -> Delay13/1
  Delay12/1 -> Out1/1
  Delay13/1 -> Delay14/1
  Delay14/1 -> Delay15/1
  Delay15/1 -> validOut/1

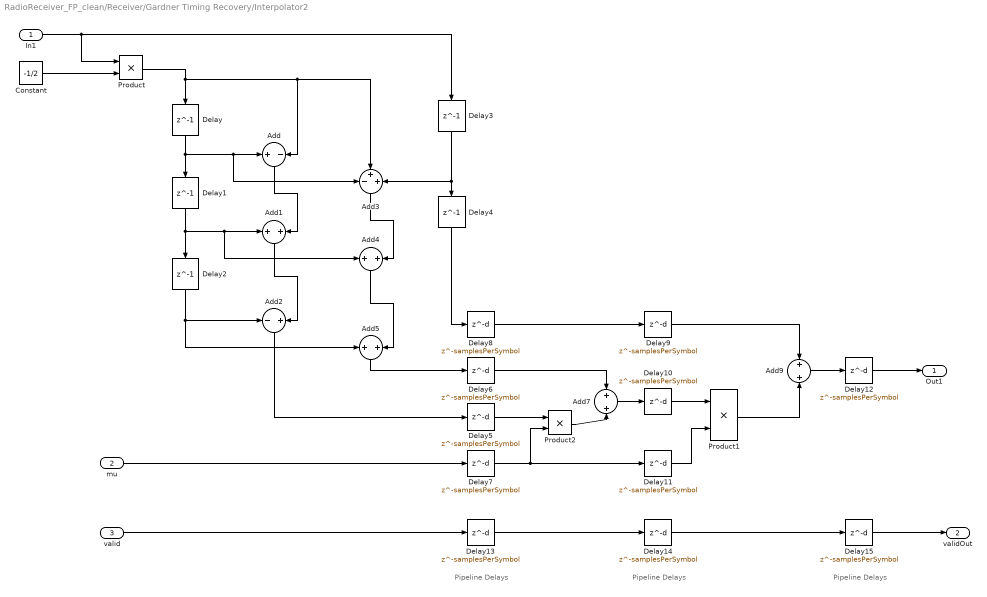
== system RadioReceiver_FP_clean/Receiver/Gardner Timing Recovery/Interpolator2 ==
  note: Pipeline Delays
  note: Pipeline Delays
  note: Pipeline Delays
  In1 : Inport  OutDataTypeStr=fixdt(1,16,13)
  mu : Inport  Port=2  OutDataTypeStr=fixdt(0,14,15)
  valid : Inport  Port=3  OutDataTypeStr=boolean
  Add : Sum  Inputs=+-  OutDataTypeStr=fixdt(1,16,15)
  Add{1,4..5,7} (4 alike) : Sum  OutDataTypeStr=fixdt(1,16,14)
  Add2 : Sum  Inputs=-+  OutDataTypeStr=fixdt(1,16,15)
  Add3 : Sum  Inputs=-++  OutDataTypeStr=fixdt(1,16,13)
  Add9 : Sum  OutDataTypeStr=fixdt(1,16,13)
  Constant : Constant  Value=-1/2  OutDataTypeStr=fixdt(1,16,16)  SampleTime=1e-06
  Delay{,1..4} (5 alike) : Delay  DelayLength=1
  Delay{5..15} (11 alike) : Delay  DelayLength=samplesPerSymbol
  Product : Product  OutDataTypeStr=fixdt(1,16,14)
  Product1 : Product  OutDataTypeStr=fixdt(1,16,14)
  Product2 : Product  OutDataTypeStr=fixdt(1,16,15)
  Out1 : Outport
  validOut : Outport  Port=2
  wires:
  In1/1 -> Delay3/1, Product/1
  Constant/1 -> Product/2
  Product/1 -> Add3/2, Add/2, Delay/1
  Delay/1 -> Add3/1, Add/1, Delay1/1
  Delay1/1 -> Add4/1, Add1/1, Delay2/1
  Add/1 -> Add1/2
  Delay2/1 -> Add5/1, Add2/1
  Add1/1 -> Add2/2
  Add3/1 -> Add4/2
  Add4/1 -> Add5/2
  Add2/1 -> Delay5/1
  mu/1 -> Delay7/1
  Add5/1 -> Delay6/1
  Product2/1 -> Add7/2
  Add9/1 -> Delay12/1
  Delay3/1 -> Add3/3, Delay4/1
  Delay4/1 -> Delay8/1
  Product1/1 -> Add9/2
  Delay5/1 -> Product2/1
  Delay6/1 -> Add7/1
  Delay7/1 -> Product2/2, Delay11/1
  Delay8/1 -> Delay9/1
  Delay9/1 -> Add9/1
  Add7/1 -> Delay10/1
  Delay10/1 -> Product1/1
  Delay11/1 -> Product1/2
  valid/1 -> Delay13/1
  Delay12/1 -> Out1/1
  Delay13/1 -> Delay14/1
  Delay14/1 -> Delay15/1
  Delay15/1 -> validOut/1

== system RadioReceiver_FP_clean/Receiver/Gardner Timing Recovery/LoopFilter ==
  e : Inport  OutDataTypeStr=fixdt(1,16,11)
  Add : Sum  OutDataTypeStr=fixdt(1,16,26)
  Add1 : Sum  OutDataTypeStr=fixdt(1,16,20)
  Delay : Delay  DelayLength=1
  Delay1 : Delay  DelayLength=1
  Intergrator Gain : Gain  Gain=IntegratorGain  OutDataTypeStr=fixdt(1,16,30)
  Proportional Gain : Gain  Gain=ProportionalGain  OutDataTypeStr=fixdt(1,16,20)
  v : Outport
  wires:
  Add/1 -> Add1/1, Delay1/1
  e/1 -> Proportional Gain/1, Intergrator Gain/1
  Intergrator Gain/1 -> Delay/1
  Delay/1 -> Add/1
  Delay1/1 -> Add/2
  Add1/1 -> v/1
  Proportional Gain/1 -> Add1/2

== system RadioReceiver_FP_clean/Receiver/Frame Sync and Decode/Barker Locate/ABS1 ==
  In1 : Inport
  Add : Sum
  Complex to Real-Imag : ComplexToRealImag
  Product : Product  OutDataTypeStr=int16
  Product1 : Product  OutDataTypeStr=int16
  Out1 : Outport
  wires:
  In1/1 -> Complex to Real-Imag/1
  Complex to Real-Imag/2 -> Product1/2, Product1/1
  Complex to Real-Imag/1 -> Product/1, Product/2
  Product/1 -> Add/1
  Product1/1 -> Add/2
  Add/1 -> Out1/1

== system RadioReceiver_FP_clean/Receiver/Frame Sync and Decode/Barker Locate/ABS2 ==
  In1 : Inport
  Add : Sum  SaturateOnIntegerOverflow=on
  Complex to Real-Imag : ComplexToRealImag
  Product : Product  OutDataTypeStr=int16
  Product1 : Product  OutDataTypeStr=int16
  Out1 : Outport
  wires:
  In1/1 -> Complex to Real-Imag/1
  Complex to Real-Imag/2 -> Product1/2, Product1/1
  Complex to Real-Imag/1 -> Product/1, Product/2
  Product/1 -> Add/1
  Product1/1 -> Add/2
  Add/1 -> Out1/1

== system RadioReceiver_FP_clean/Receiver/Frame Sync and Decode/Barker Locate/HDL Opt Complex FIR ==
  In1 : Inport
  validIn : Inport  Port=2
  Add : Sum  AccumDataTypeStr=fixdt(1,16,0)
  Discrete FIR Filter HDL Optimized : dsphdlfiltering/Discrete FIR Filter HDL Optimized  Numerator=real(Taps)  Sharing=off  SharingFactor=2  SimulateUsing=Code generation  roundingMode=Floor  overflowMode=off  CoefficientsDataTypeStr=Inherit: Same word length as input  CoefficientsMin=[]  CoefficientsMax=[]  OutputDataTypeStr=fixdt(1,15,0)  OutputMin=[]  OutputMax=[]  ValidInPort=on  ReadyPort=off
      settings: SourceProductName=DSP System Toolbox  SourceProductBaseCode=DS
  Discrete FIR Filter HDL Optimized1 : dsphdlfiltering/Discrete FIR Filter HDL Optimized  Numerator=imag(Taps)  Sharing=off  SharingFactor=2  SimulateUsing=Code generation  roundingMode=Floor  overflowMode=off  CoefficientsDataTypeStr=Inherit: Same word length as input  CoefficientsMin=[]  CoefficientsMax=[]  OutputDataTypeStr=fixdt(1,15,0)  OutputMin=[]  OutputMax=[]  ValidInPort=on  ReadyPort=off
      settings: SourceProductName=DSP System Toolbox  SourceProductBaseCode=DS
  Logical Operator : Logic  AllPortsSameDT=off  OutDataTypeStr=boolean
  Out1 : Outport
  validOut : Outport  Port=2
  wires:
  In1/1 -> Discrete FIR Filter HDL Optimized1/1, Discrete FIR Filter HDL Optimized/1
  Discrete FIR Filter HDL Optimized/1 -> Add/1
  Add/1 -> Out1/1
  Logical Operator/1 -> validOut/1
  Discrete FIR Filter HDL Optimized/2 -> Logical Operator/1
  Discrete FIR Filter HDL Optimized1/2 -> Logical Operator/2
  Discrete FIR Filter HDL Optimized1/1 -> Add/2
  validIn/1 -> Discrete FIR Filter HDL Optimized1/2, Discrete FIR Filter HDL Optimized/2

== system RadioReceiver_FP_clean/Receiver/Frame Sync and Decode/Barker Locate/Measure Phase Ambiguity ==
  In1 : Inport  OutDataTypeStr=int16
  trigger : Inport  Port=2
  Discrete FIR Filter1 : DiscreteFir  Coefficients=exp(-j*pi/2).*xPreambleSeq(end:-1:1).'  AccumDataTypeStr=Inherit: Same as product output  OutDataTypeStr=int16
  Discrete FIR Filter2 : DiscreteFir  Coefficients=xPreambleSeq(end:-1:1).'  AccumDataTypeStr=Inherit: Same as product output  OutDataTypeStr=int16
  Discrete FIR Filter3 : DiscreteFir  Coefficients=exp(-j*pi).*xPreambleSeq(end:-1:1).'  AccumDataTypeStr=Inherit: Same as product output  OutDataTypeStr=int16
  Discrete FIR Filter4 : DiscreteFir  Coefficients=exp(-j*pi*3/2).*xPreambleSeq(end:-1:1).'  AccumDataTypeStr=Inherit: Same as product output  OutDataTypeStr=int16
  Find Max and Set Output Shift : Subsystem
  Out1 : Outport  InitialOutput=0
  wires:
  In1/1 -> Discrete FIR Filter4/1, Discrete FIR Filter3/1, Discrete FIR Filter1/1, Discrete FIR Filter2/1
  Discrete FIR Filter2/1 -> Find Max and Set Output Shift/1(In1)
  Discrete FIR Filter1/1 -> Find Max and Set Output Shift/2(In2)
  Discrete FIR Filter3/1 -> Find Max and Set Output Shift/3(In4)
  Discrete FIR Filter4/1 -> Find Max and Set Output Shift/4(In5)
  trigger/1 -> Find Max and Set Output Shift/Enable
  Find Max and Set Output Shift/1(Out1) -> Out1/1

== system RadioReceiver_FP_clean/Receiver/Frame Sync and Decode/Barker Locate/Measure Phase Ambiguity1 ==
  data : Inport  OutDataTypeStr=int16
  trigger : Inport  Port=2
  validIn : Inport  Port=3
  Find Max and Set Output Shift : Subsystem
  HDL Opt Complex FIR4 : Subsystem  mask{Taps=xPreambleSeq(end:-1:1).'}
  HDL Opt Complex FIR5 : Subsystem  mask{Taps=exp(-j*pi/2).*xPreambleSeq(end:-1:1).'}
  HDL Opt Complex FIR6 : Subsystem  mask{Taps=exp(-j*pi).*xPreambleSeq(end:-1:1).'}
  HDL Opt Complex FIR7 : Subsystem  mask{Taps=exp(-j*pi*3/2).*xPreambleSeq(end:-1:1).'}
  Logical Operator : Logic  Inputs=5  AllPortsSameDT=off  OutDataTypeStr=boolean
  PA : Outport  InitialOutput=0
  wires:
  data/1 -> HDL Opt Complex FIR4/1(In1), HDL Opt Complex FIR5/1(In1), HDL Opt Complex FIR7/1(In1), HDL Opt Complex FIR6/1(In1)
  HDL Opt Complex FIR4/1(Out1) -> Find Max and Set Output Shift/1(In1)
  HDL Opt Complex FIR5/1(Out1) -> Find Max and Set Output Shift/2(In2)
  HDL Opt Complex FIR6/1(Out1) -> Find Max and Set Output Shift/3(In4)
  HDL Opt Complex FIR7/1(Out1) -> Find Max and Set Output Shift/4(In5)
  Find Max and Set Output Shift/1(Out1) -> PA/1
  validIn/1 -> HDL Opt Complex FIR4/2(validIn), HDL Opt Complex FIR5/2(validIn), HDL Opt Complex FIR7/2(validIn), HDL Opt Complex FIR6/2(validIn)
  HDL Opt Complex FIR4/2(validOut) -> Logical Operator/1
  HDL Opt Complex FIR5/2(validOut) -> Logical Operator/2
  HDL Opt Complex FIR6/2(validOut) -> Logical Operator/3
  HDL Opt Complex FIR7/2(validOut) -> Logical Operator/4
  Logical Operator/1 -> Find Max and Set Output Shift/Enable
  trigger/1 -> Logical Operator/5

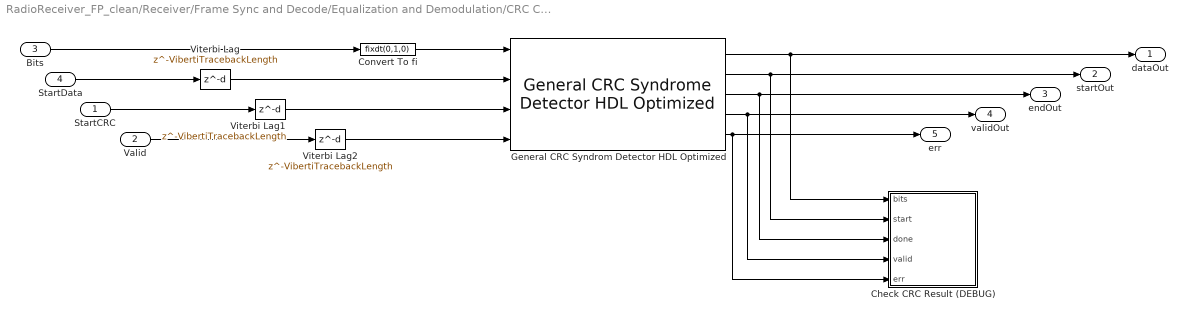
== system RadioReceiver_FP_clean/Receiver/Frame Sync and Decode/Equalization and Demodulation/CRC Check ==
  StartCRC : Inport
  Valid : Inport  Port=2
  Bits : Inport  Port=3
  StartData : Inport  Port=4
  Check CRC Result (DEBUG) : MATLAB Function  TreatAsAtomicUnit=on
  Convert To fi : DataTypeConversion  OutDataTypeStr=fixdt(0,1,0)  SaturateOnIntegerOverflow=on
  General CRC Syndrom Detector HDL Optimized : commcrc2/General CRC Syndrome Detector HDL Optimized  Polynomial=crc32Poly  InitialState=0  DirectMethod=off  ReflectInput=off  ReflectCRCChecksum=off  FinalXORValue=0  SimulateUsing=Code generation
      settings: SourceProductName=Communications System Toolbox  SourceProductBaseCode=CM
  Viterbi Lag : Delay  DelayLength=VibertiTracebackLength
  Viterbi Lag1 : Delay  DelayLength=VibertiTracebackLength
  Viterbi Lag2 : Delay  DelayLength=VibertiTracebackLength
  dataOut : Outport
  startOut : Outport  Port=2
  endOut : Outport  Port=3
  validOut : Outport  Port=4
  err : Outport  Port=5
  wires:
  StartCRC/1 -> Viterbi Lag1/1
  Valid/1 -> Viterbi Lag2/1
  StartData/1 -> Viterbi Lag/1
  Bits/1 -> Convert To fi/1
  General CRC Syndrom Detector HDL Optimized/1 -> Check CRC Result (DEBUG)/1(bits), dataOut/1
  General CRC Syndrom Detector HDL Optimized/3 -> Check CRC Result (DEBUG)/3(done), endOut/1
  General CRC Syndrom Detector HDL Optimized/4 -> Check CRC Result (DEBUG)/4(valid), validOut/1
  General CRC Syndrom Detector HDL Optimized/5 -> Check CRC Result (DEBUG)/5(err), err/1
  General CRC Syndrom Detector HDL Optimized/2 -> Check CRC Result (DEBUG)/2(start), startOut/1
  Convert To fi/1 -> General CRC Syndrom Detector HDL Optimized/1
  Viterbi Lag/1 -> General CRC Syndrom Detector HDL Optimized/2
  Viterbi Lag2/1 -> General CRC Syndrom Detector HDL Optimized/4
  Viterbi Lag1/1 -> General CRC Syndrom Detector HDL Optimized/3

== system RadioReceiver_FP_clean/Receiver/Frame Sync and Decode/Equalization and Demodulation/DFE ==
  note: Generate training sequence when barker is found
  Trigger : Inport
  data : Inport  Port=2
  Delay data so DFE can reset : Delay  DelayLength=1
  Delay ref so DFE can reset : Delay  DelayLength=1
  Equalizer : MATLAB Function  TreatAsAtomicUnit=on
  PN Sequence Generator : commseqgen3/PN Sequence Generator  poly='z^3 + z^2 + 1'  ini_sta=[0 0 1]  outBitMaskSource=Dialog parameter  shift=0  outVarSiz=off  maxOutSizeMode=Dialog parameter  maxOutSize=[10 1]  Ts=1/(RadioSampleRate*1)  sampPerFrame=1  reset=on  bitPackedOutputs=on  outDataType=Smallest unsigned integer  numPackedBits=2  bitPackDataSigned=off  bitPackedOutDType=Smallest integer
      settings: SourceProductName=Communications System Toolbox
  Packeted To Unpacked : Subsystem
  QPSK Modulator Baseband : commdigbbndpm3/QPSK Modulator Baseband  InType=Bit  Enc=Binary  Ph=pi/4  outDtype=Fixed-point  outWordLen=16  outUDDataType=sfix(16)  outFracLenMode=User-defined  outFracLen=14  outDataTypeStr=fixdt(1,16,14)  outLastDataTypeStr=fixdt(1,16,14)
  dataEQed : Outport
  wires:
  Equalizer/1(eqOut) -> dataEQed/1
  Trigger/1 -> Equalizer/1(trigger), PN Sequence Generator/1
  data/1 -> Delay data so DFE can reset/1
  PN Sequence Generator/1 -> Packeted To Unpacked/1(In1)
  Packeted To Unpacked/1(Out1) -> QPSK Modulator Baseband/1
  QPSK Modulator Baseband/1 -> Delay ref so DFE can reset/1
  Delay data so DFE can reset/1 -> Equalizer/2(data)
  Delay ref so DFE can reset/1 -> Equalizer/3(trainingSymbol)

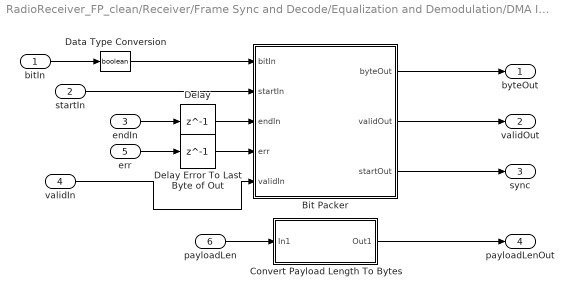
== system RadioReceiver_FP_clean/Receiver/Frame Sync and Decode/Equalization and Demodulation/DMA Interface ==
  bitIn : Inport
  startIn : Inport  Port=2
  endIn : Inport  Port=3
  validIn : Inport  Port=4
  err : Inport  Port=5
  payloadLen : Inport  Port=6
  Bit Packer : MATLAB Function  TreatAsAtomicUnit=on
  Convert Payload Length To Bytes : Subsystem
  Data Type Conversion : DataTypeConversion  OutDataTypeStr=boolean
  Delay : Delay  DelayLength=1
  Delay Error To Last Byte of Out : Delay  DelayLength=1
  byteOut : Outport
  validOut : Outport  Port=2
  sync : Outport  Port=3
  payloadLenOut : Outport  Port=4
  wires:
  bitIn/1 -> Data Type Conversion/1
  Delay/1 -> Bit Packer/3(endIn)
  Delay Error To Last Byte of Out/1 -> Bit Packer/4(err)
  Bit Packer/2(validOut) -> validOut/1
  Bit Packer/3(startOut) -> sync/1
  Bit Packer/1(byteOut) -> byteOut/1
  err/1 -> Delay Error To Last Byte of Out/1
  validIn/1 -> Bit Packer/5(validIn)
  endIn/1 -> Delay/1
  startIn/1 -> Bit Packer/2(startIn)
  Data Type Conversion/1 -> Bit Packer/1(bitIn)
  payloadLen/1 -> Convert Payload Length To Bytes/1(In1)
  Convert Payload Length To Bytes/1(Out1) -> payloadLenOut/1

== system RadioReceiver_FP_clean/Receiver/Frame Sync and Decode/Equalization and Demodulation/Descramble and Decode ==
  Bits : Inport
  reset : Inport  Port=2
  Enable : EnablePort
  2 Bit Descrambler : Subsystem  mask{polynom=[1 1 0 1 0 1 0 1], initstate=[0 1 0 0 0 1 0]}
      mask prompts: polynom "Polynomial"; initstate "Inital State"
      mask Display: fprintf('HDL Descrambler')
  Demux : Demux  Commented=on  Outputs=2
  Enabled Subsystem : Subsystem  Commented=on  TreatAsAtomicUnit=on
  Find packet tail and check CRC (DEBUG ONLY) : MATLAB Function  Commented=on  TreatAsAtomicUnit=on
  "Pipeline Delay (REMOVE BEFORE SYNTH, ONLY FOR SIMULATION)" : Delay  DelayLength=20
  Terminator : Terminator  Commented=on
  Viterbi Decoder : commcnvcod2/Viterbi Decoder  trellis=poly2trellis(7, [171 133])  isPunctured=off  punctureVector=[1; 1; 0; 1; 0; 1]  erasures=off  dectype=Hard decision  nsdecb=4  runSigValErrCheck=off  tbdepth=VibertiTracebackLength-20  opmode=Continuous  reset=on  delayedResetAction=on  smWordLength=16  outDataType=boolean
      settings: SourceProductName=Communications System Toolbox  SourceProductBaseCode=CM
  Decoded Bits : Outport  InitialOutput=0
  wires:
  reset/1 -> 2 Bit Descrambler/2(reset), Viterbi Decoder/2
  Bits/1 -> 2 Bit Descrambler/1(u1)
  Demux/2 -> Terminator/1
  Find packet tail and check CRC (DEBUG ONLY)/1(enable) -> Enabled Subsystem/Enable
  Find packet tail and check CRC (DEBUG ONLY)/2(crcCase) -> Enabled Subsystem/1(In1)
  2 Bit Descrambler/1(y1) -> Demux/1, Viterbi Decoder/1
  Viterbi Decoder/1 -> "Pipeline Delay (REMOVE BEFORE SYNTH, ONLY FOR SIMULATION)"/1
  "Pipeline Delay (REMOVE BEFORE SYNTH, ONLY FOR SIMULATION)"/1 -> Decoded Bits/1, Find packet tail and check CRC (DEBUG ONLY)/1(u)

== system RadioReceiver_FP_clean/Receiver/Gardner Timing Recovery/Gardner TED Blocks/Imag Error ==
  data : Inport
  strobe sum : Inport  Port=2
  Delay : Delay  DelayLength=1
  Product1 : Product  OutDataTypeStr=fixdt(1,16,13)
  Sub : Sum  Inputs=+-  AccumDataTypeStr=fixdt(1,16,13)
  TED Buffer Update1 : Subsystem
  Out1 : Outport
  wires:
  Product1/1 -> Out1/1
  Sub/1 -> Product1/2
  data/1 -> Sub/2, Delay/1
  strobe sum/1 -> TED Buffer Update1/2(strobe sum)
  TED Buffer Update1/2(oldest) -> Sub/1
  Delay/1 -> TED Buffer Update1/1(new data)
  TED Buffer Update1/1(Middle Indx) -> Product1/1
